simulink model "MotorXploer"  (R2025b)
settings: Solver=FixedStepAuto  StartTime=0.0  StopTime=inf  FixedStep=0.001  RelTol=1e-3  EnableMultiTasking=on
values from neighbouring files (symbols this model uses):
  bw_den = [1, A2 / A1, A3 / A1]    [Lab1_motor_params_student.m]
  bw_num = [(Km * dt2) / A1, 0, 0]    [Lab1_motor_params_student.m]
  dt = 0.01    [Lab1_motor_params_student.m]    (also in comport.m = 0.002)
  fw_den = [1, fw_termW1, fw_termW2]    [Lab1_motor_params_student.m]
  fw_num = [0, 0, fw_termV]    [Lab1_motor_params_student.m]
  motor_B = 8.84E-05    (= 8.84e-05)    [Lab1_motor_params_student.m]
  motor_B_Chirp = 4.18E-04    (= 0.000418)    [Lab1_motor_params_student.m]
  motor_B_Ramp = 1.07E-04    (= 0.000107)    [Lab1_motor_params_student.m]
  motor_B_Sin2Pi = 7.21e-05    [Lab1_motor_params_student.m]
  motor_B_SinPi = 1.55E-04    (= 0.000155)    [Lab1_motor_params_student.m]
  motor_B_SinPi_2 = 7.21E-05    (= 7.21e-05)    [Lab1_motor_params_student.m]
  motor_B_Stair = 6.12303E-05    (= 6.12303e-05)    [Lab1_motor_params_student.m]
  motor_Eff = 0.99866    [Lab1_motor_params_student.m]
  motor_Eff_Chirp = 0.992383333    [Lab1_motor_params_student.m]
  motor_Eff_Ramp = 0.973136667    [Lab1_motor_params_student.m]
  motor_Eff_Sin2Pi = 9.99e-01    (= 0.999)    [Lab1_motor_params_student.m]
  motor_Eff_SinPi = 0.99474    [Lab1_motor_params_student.m]
  motor_Eff_SinPi_2 = 0.999073333    [Lab1_motor_params_student.m]
  motor_Eff_Stair = 0.999076667    [Lab1_motor_params_student.m]
  motor_J = 1.46E-05    (= 1.46e-05)    [Lab1_motor_params_student.m]
  motor_J_Chirp = 1.12E-06    (= 1.12e-06)    [Lab1_motor_params_student.m]
  motor_J_Ramp = 0.000341863    [Lab1_motor_params_student.m]
  motor_J_Sin2Pi = 1.27e-05    [Lab1_motor_params_student.m]
  motor_J_SinPi = 1.28492E-05    (= 1.28492e-05)    [Lab1_motor_params_student.m]
  motor_J_SinPi_2 = 1.26993E-05    (= 1.26993e-05)    [Lab1_motor_params_student.m]
  motor_J_Stair = 1.35E-05    (= 1.35e-05)    [Lab1_motor_params_student.m]
  motor_Ke = 0.041524    [Lab1_motor_params_student.m]
  motor_Ke_Chirp = 0.070106333    [Lab1_motor_params_student.m]
  motor_Ke_Ramp = 0.037761333    [Lab1_motor_params_student.m]
  motor_Ke_Sin2Pi = 4.52e-02    (= 0.0452)    [Lab1_motor_params_student.m]
  motor_Ke_SinPi = 0.030033333    [Lab1_motor_params_student.m]
  motor_Ke_SinPi_2 = 0.045154    [Lab1_motor_params_student.m]
  motor_Ke_Stair = 0.044075    [Lab1_motor_params_student.m]
  motor_L = 0.002919699    [Lab1_motor_params_student.m]
  motor_R = 3.824    [Lab1_motor_params_student.m]
  tz_den = [1, B2 / B1, B3 / B1]    [Lab1_motor_params_student.m]
  tz_num = [(Km * dt2) / B1, (2 * Km * dt2) / B1, (Km * dt2) / B1]    [Lab1_motor_params_student.m]
undefined symbols (not defined in the file or in its folder): Blocking, dspblkCoreblockFVToolHelper, gcbh, LF, Non
libraries: simulink x31, amg_usbconverter_n_connect_lib x3
settings Model: Creator=beamk  LastModifiedBy=gonth
settings SolverCC: AutoInsertRateTranBlk=on
settings OptimizationCC: DefaultParameterBehavior=Inlined  EnhancedBackFolding=on  PassReuseOutputArgsAs=Individual arguments  ZeroExternalMemoryAtStartup=off  ZeroInternalMemoryAtStartup=off  MaxStackSize=64  OptimizeBlockOrder=speed  DifferentSizesBufferReuse=on  OptimizationCustomize=off  EfficientTunableParamExpr=on
settings DebuggingCC: ParameterTunabilityLossMsg=error
settings HardwareCC: ProdBitPerPointer=32.0  ProdBitPerSizeT=32.0  ProdBitPerPtrDiffT=32.0  ProdLargestAtomicInteger=Long  ProdLargestAtomicFloat=Double  ProdWordSize=32.0  ProdLongLongMode=on  ProdHWDeviceType=ARM Compatible->ARM Cortex-M
settings SFSimCC: MATLABDynamicMemAlloc=off
settings RTWCC: SystemTargetFile=ert.tlc  HardwareBoard=STM32G4xx Based  TemplateMakefile=ert_default_tmf  Toolchain=Armclang Compiler  Description=Embedded Coder
settings CodeAppCC: ForceParamTrailComments=on  IgnoreCustomStorageClasses=off  OperatorAnnotations=on  SimulinkDataObjDesc=on  SFDataObjDesc=on  InsertBlockDesc=on
settings ERTTargetCC: ExtModeTransport=3.0  ExtModeStaticAlloc=on  ExtModeStaticAllocSize=2048.0  ExtModeMexFile=ext_xcp  ExtModeIntrfLevel=Level2 - Open  TargetLangStandard=C99 (ISO)  CodeReplacementLibrary=ARM Cortex-M

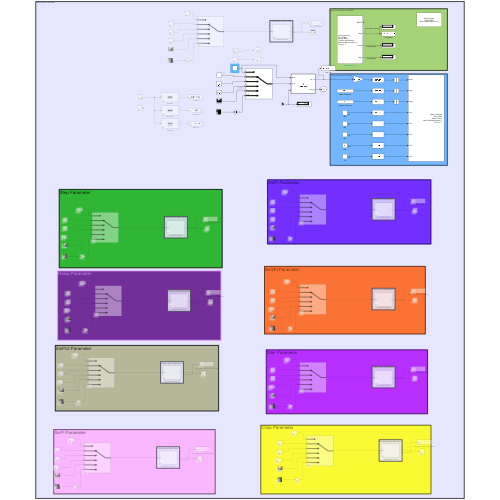
[thumbnail: Simulink's stored preview of the top-level diagram]
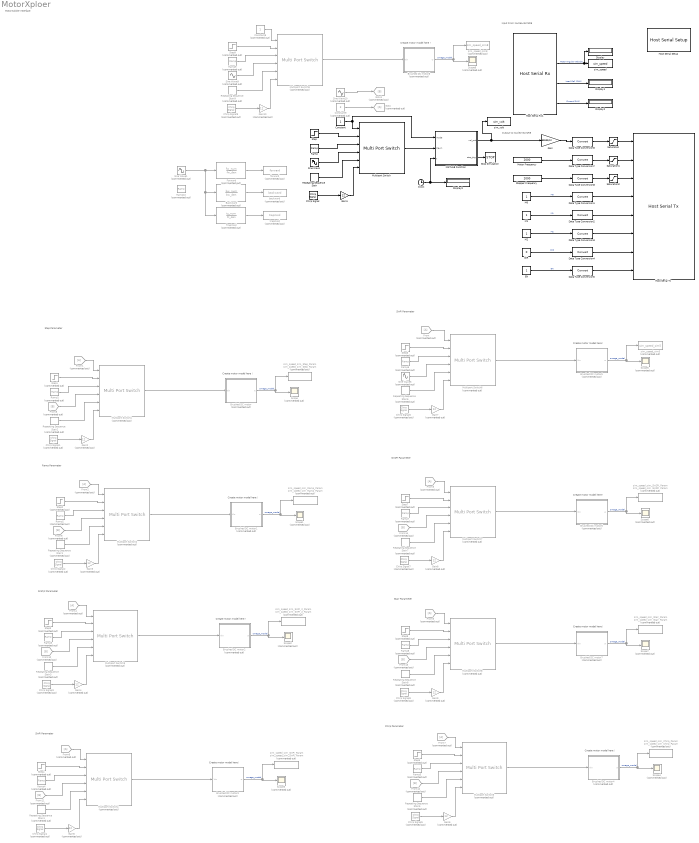
== system MotorXploer ==
  note: Output to Nucleo-G474RE
  note: Input From Nucleo-G474RE
  note: MotorXploler Interface
  note: Create motor model here !
  note: Create motor model here !
  note: Create motor model here !
  note: Create motor model here !
  note: Create motor model here !
  note: Create motor model here !
  note: Create motor model here !
  note: Create motor model here !
  note: Create motor model here !
  note: Step Parameter
  note: Ramp Parameter
  note: SinPi/2 Parameter
  note: SinPi Parameter
  note: SinPi Parameter
  note: Sin2Pi Parameter
  note: Stair Parameter
  note: Chirp Parameter
  Backward : DiscreteFilter  Commented=on  LoadFcn=dspblkCoreblockFVToolHelper(gcbh,'load');  Numerator=bw_num  Denominator=bw_den
      settings: CopyFcn=dspblkCoreblockFVToolHelper(gcbh,'copy');  DeleteFcn=dspblkCoreblockFVToolHelper(gcbh,'close');  ModelCloseFcn=dspblkCoreblockFVToolHelper(gcbh,'close');  PreSaveFcn=dspblkCoreblockFVToolHelper(gcbh,'presave');  PostSaveFcn=dspblkCoreblockFVToolHelper(gcbh,'postsave');  CloseFcn=dspblkCoreblockFVToolHelper(gcbh,'close');
  Brushed DC motor : Subsystem  Commented=on
  Brushed DC motor1 : Subsystem  Commented=on
  Brushed DC motor2 : Subsystem  Commented=on
  Brushed DC motor3 : Subsystem  Commented=on
  Brushed DC motor4 : Subsystem  Commented=on
  Brushed DC motor5 : Subsystem  Commented=on
  Brushed DC motor6 : Subsystem  Commented=on
  Brushed DC motor7 : Subsystem  Commented=on
  Brushed DC motor8 : Subsystem  Commented=on
  Chirp Signal : simulink/Sources/Chirp Signal  f1=0.1  T=30  f2=1
  Chirp Signal{1..9} (9 alike) : simulink/Sources/Chirp Signal  Commented=on  f1=0.1  T=30  f2=1
  Clock : Clock
  Constant : Constant
  Constant6 : Constant  Commented=on
  Constant9 : Constant  Commented=on  Value=3
  DIR : Constant  Value=0
  Data Type Conversion{1..8} (8 alike) : DataTypeConversion  SaturateOnIntegerOverflow=off  RndMeth=Floor
  Display{,1..3} (4 alike) : Display
  EN : Constant
  Forward : DiscreteFilter  Commented=on  LoadFcn=dspblkCoreblockFVToolHelper(gcbh,'load');  Numerator=fw_num  Denominator=fw_den
      settings: CopyFcn=dspblkCoreblockFVToolHelper(gcbh,'copy');  DeleteFcn=dspblkCoreblockFVToolHelper(gcbh,'close');  ModelCloseFcn=dspblkCoreblockFVToolHelper(gcbh,'close');  PreSaveFcn=dspblkCoreblockFVToolHelper(gcbh,'presave');  PostSaveFcn=dspblkCoreblockFVToolHelper(gcbh,'postsave');  CloseFcn=dspblkCoreblockFVToolHelper(gcbh,'close');
  From{,1..7} (8 alike) : From  Commented=on
  From{8..14} (7 alike) : From  Commented=on  GotoTag=B
  Gain : Gain  Gain=65535/12
  Gain1 : Gain  Gain=12
  Gain{2..10} (9 alike) : Gain  Commented=on  Gain=12
  Goto : Goto  Commented=on
  Goto1 : Goto  Commented=on  GotoTag=B
  Host Serial Rx1 : amg_usbconverter_n_connect_lib/Host Serial Rx  conf=rx  port=<auto>  baudrate=2000000  databits=8  parity=None  stopbit=1  flowcontrol=None  transfer=Non-Blocking  timeout=5  packetmode=Binary  enableinitialvalues=off  initialvalues=[]  binheader='25'  binterminator='4E'  porttype_double=0  porttype_single=3  porttype_int8=0  porttype_uint8=0  porttype_int16=0  porttype_uint16=0  porttype_int32=0  porttype_uint32=0  asciiformat='%f,%f,%d,%d'  rx_asciiterminator="LF (0x0A - \"\\n\")"  tx_asciiterminator="CRLF (0x0D 0x0A - \"\\r\\n\")"  sampletime=-1  enablecustomportlabel=off  cinputportlabel=0  coutputportlabel=A  portpinstr=0  blockid=HostSerialRx1  inputporttype=[]  inputportwidth=[]  inputportlabel={}  outputporttype=[3 1 1 1]  outputportwidth=[1 1 1 1]  outputportlabel={'READY','single','single','single'}  compat=0  optionstring=[]  autoport='COM5'
  Host Serial Setup : amg_usbconverter_n_connect_lib/Host Serial Setup  conf=setup  port=<auto>  baudrate=2000000  databits=8  parity=None  stopbit=1  flowcontrol=None  transfer=Blocking  timeout=2  packetmode=Binary  initialvalues=[]  binheader='7E 7E'  binterminator='03 03'  porttype_double=0  porttype_single=1  porttype_int8=0  porttype_uint8=0  porttype_int16=0  porttype_uint16=0  porttype_int32=0  porttype_uint32=2  asciiformat='%d %u %x'  rx_asciiterminator="CRLF (0x0D 0x0A - \"\\r\\n\")"  tx_asciiterminator="CRLF (0x0D 0x0A - \"\\r\\n\")"  sampletime=-1  enablecustomportlabel=off  cinputportlabel=0  coutputportlabel=A  portpinstr=0  blockid=HostSerialSetup  inputporttype=[]  inputportwidth=[]  inputportlabel={}  outputporttype=[]  outputportwidth=[]  outputportlabel={}  compat=0  optionstring=[]  autoport='COM5'
  Host Serial Tx : amg_usbconverter_n_connect_lib/Host Serial Tx  conf=tx  port=<auto>  baudrate=2000000  databits=8  parity=None  stopbit=1  flowcontrol=None  transfer=Blocking  timeout=2  packetmode=Binary  initialvalues=[]  binheader='25'  binterminator='4E'  porttype_double=0  porttype_single=3  porttype_int8=0  porttype_uint8=0  porttype_int16=5  porttype_uint16=0  porttype_int32=0  porttype_uint32=0  asciiformat='%d,%f'  rx_asciiterminator="CRLF (0x0D 0x0A - \"\\r\\n\")"  tx_asciiterminator="CRLF (0x0D 0x0A - \"\\r\\n\")"  sampletime=-1  enablecustomportlabel=off  cinputportlabel=0  coutputportlabel=A  portpinstr=0  blockid=HostSerialTx  inputporttype=[1 1 1 4 4 4 4 4]  inputportwidth=[1 1 1 1 1 1 1 1]  inputportlabel={'single','single','single','int16','int16','int16','int16','int16'}  outputporttype=[]  outputportwidth=[]  outputportlabel={}  compat=0  optionstring=[]  autoport='COM5'
      settings: SourceProductName=aMG USB Converter N
  M0 : Constant
  M1 : Constant
  M2 : Constant
  MATLAB Function : MATLAB Function  TreatAsAtomicUnit=on
  Motor Frequency : Constant  Value=2000  OutDataTypeStr=single
  Multiport Switch : MultiPortSwitch  Inputs=5  SaturateOnIntegerOverflow=off  InputSameDT=off
  Multiport Switch{1..9} (9 alike) : MultiPortSwitch  Commented=on  Inputs=5  SaturateOnIntegerOverflow=off  InputSameDT=off
  Ramp : simulink/Sources/Ramp  slope=1  start=1  InitialOutput=0
  Ramp{1..9} (9 alike) : simulink/Sources/Ramp  Commented=on  slope=.48  start=0  InitialOutput=0
  Ramp10 : simulink/Sources/Ramp  Commented=on  slope=1  start=1  InitialOutput=0
  Repeating Sequence Stair : simulink/Sources/Repeating Sequence Stair  OutValues="[0  3 0 6 0 9 0 12].'"  tsamp=2.778  OutMin=[]  OutMax=[]  OutDataTypeStr=double  OutputDataTypeScalingMode=double  OutDataType=fixdt(0,8)  ConRadixGroup=Best Precision: Vector-wise  OutScaling=2^-12
  Repeating Sequence Stair{1..9} (9 alike) : simulink/Sources/Repeating Sequence Stair  Commented=on  OutValues=[0 3 0 6 0 9 0 12].'  tsamp=2.778  OutMin=[]  OutMax=[]  OutDataTypeStr=double  OutputDataTypeScalingMode=double  OutDataType=fixdt(0,8)  ConRadixGroup=Best Precision: Vector-wise  OutScaling=2^-12
  Saturation : Saturate  UpperLimit=65535  LowerLimit=-65535
  Saturation1 : Saturate  UpperLimit=20000  LowerLimit=0
  Saturation2 : Saturate  UpperLimit=inf  LowerLimit=0
  Scope{,1..8} (9 alike) : Scope  Commented=on
      Scope settings: ActiveDisplayYMinimum=-7.4641136436048834  ActiveDisplayYMaximum=11.461850298961346
      Scope1 settings: ActiveDisplayYMinimum=-7.4641136436048834  ActiveDisplayYMaximum=11.461850298961346
      Scope2 settings: ActiveDisplayYMinimum=-7.4641136436048834  ActiveDisplayYMaximum=11.461850298961346  DataLoggingVariableName=ScopeData2
      Scope3 settings: ActiveDisplayYMinimum=-7.4641136436048834  ActiveDisplayYMaximum=11.461850298961346  DataLoggingVariableName=ScopeData3
      Scope4 settings: ActiveDisplayYMinimum=-7.4641136436048834  ActiveDisplayYMaximum=11.461850298961346  DataLoggingVariableName=ScopeData4
      Scope5 settings: ActiveDisplayYMinimum=-7.4641136436048834  ActiveDisplayYMaximum=11.461850298961346  DataLoggingVariableName=ScopeData5
      Scope6 settings: ActiveDisplayYMinimum=-7.4641136436048834  ActiveDisplayYMaximum=11.461850298961346  DataLoggingVariableName=ScopeData6
      Scope7 settings: ActiveDisplayYMinimum=-7.4641136436048834  ActiveDisplayYMaximum=11.461850298961346  DataLoggingVariableName=ScopeData7
      Scope8 settings: ActiveDisplayYMinimum=-7.4641136436048834  ActiveDisplayYMaximum=11.461850298961346  DataLoggingVariableName=ScopeData8
  Sine Wave : Sin  Amplitude=12  Frequency=pi*2  SampleTime=0
  Sine Wave1 : Sin  Commented=on  Amplitude=12  Frequency=pi*2  SampleTime=dt
  Sine Wave10 : Sin  Commented=on  Amplitude=12  Frequency=pi*2  SampleTime=0
  Sine Wave6 : Sin  Commented=on  Amplitude=12  Frequency=2*pi  SampleTime=0
  Sine Wave9 : Sin  Commented=on  Amplitude=12  Frequency=2*pi  SampleTime=0
  Step : Step  After=12  SampleTime=0
  Step{1..9} (9 alike) : Step  Commented=on  After=12  SampleTime=0
  Stepper Frequency : Constant  Value=2000  OutDataTypeStr=single
  Stop Simulation : Stop
  Trapizoid : DiscreteFilter  Commented=on  LoadFcn=dspblkCoreblockFVToolHelper(gcbh,'load');  Numerator=tz_num  Denominator=tz_den
      settings: CopyFcn=dspblkCoreblockFVToolHelper(gcbh,'copy');  DeleteFcn=dspblkCoreblockFVToolHelper(gcbh,'close');  ModelCloseFcn=dspblkCoreblockFVToolHelper(gcbh,'close');  PreSaveFcn=dspblkCoreblockFVToolHelper(gcbh,'presave');  PostSaveFcn=dspblkCoreblockFVToolHelper(gcbh,'postsave');  CloseFcn=dspblkCoreblockFVToolHelper(gcbh,'close');
  backward : ToWorkspace  Commented=on  VariableName=backward  SaveFormat=Timeseries  SampleTime=-1
  forward : ToWorkspace  Commented=on  VariableName=forward  SaveFormat=Timeseries  SampleTime=-1
  sim_speed : ToWorkspace  VariableName=sim_speed  SaveFormat=Timeseries  SampleTime=-1
  sim_speed_sim5 : ToWorkspace  Commented=on  VariableName=sim_speed_sim5  SaveFormat=Timeseries  SampleTime=-1
  sim_speed_sim8 : ToWorkspace  Commented=on  VariableName=sim_speed_sim8  SaveFormat=Timeseries  SampleTime=-1
  sim_speed_sim_Chirp_Param : ToWorkspace  Commented=on  VariableName=sim_speed_sim_Chirp_Param  SaveFormat=Timeseries  SampleTime=-1
  sim_speed_sim_Ramp_Param : ToWorkspace  Commented=on  VariableName=sim_speed_sim_Ramp_Param  SaveFormat=Timeseries  SampleTime=-1
  sim_speed_sim_Sin2Pi_Param : ToWorkspace  Commented=on  VariableName=sim_speed_sim_Sin2Pi_Param  SaveFormat=Timeseries  SampleTime=-1
  sim_speed_sim_SinPi_2_Param : ToWorkspace  Commented=on  VariableName=sim_speed_sim_SinPi_2_Param  SaveFormat=Timeseries  SampleTime=-1
  sim_speed_sim_SinPi_Param : ToWorkspace  Commented=on  VariableName=sim_speed_sim_SinPi_Param  SaveFormat=Timeseries  SampleTime=-1
  sim_speed_sim_Stair_Param : ToWorkspace  Commented=on  VariableName=sim_speed_sim_Stair_Param  SaveFormat=Timeseries  SampleTime=-1
  sim_speed_sim_Step_Param : ToWorkspace  Commented=on  VariableName=sim_speed_sim_Step_Param  SaveFormat=Timeseries  SampleTime=-1
  sim_volt : ToWorkspace  VariableName=sim_volt  SaveFormat=Timeseries  SampleTime=-1
  trapizoid : ToWorkspace  Commented=on  VariableName=trapizoid  SaveFormat=Timeseries  SampleTime=-1
  wires:
  Host Serial Rx1/2 -> sim_speed/1, Display/1  "Motor Angular Velocity"
  Host Serial Rx1/3 -> Display1/1  "Load Cell (PA0)"
  M0/1 -> Data Type Conversion1/1  "M0"
  EN/1 -> Data Type Conversion5/1  "EN"
  DIR/1 -> Data Type Conversion4/1  "DIR"
  M1/1 -> Data Type Conversion2/1  "M1"
  M2/1 -> Data Type Conversion3/1  "M2"
  Motor Frequency/1 -> Data Type Conversion7/1
  Stepper Frequency/1 -> Data Type Conversion8/1
  Data Type Conversion1/1 -> Host Serial Tx/4
  Data Type Conversion2/1 -> Host Serial Tx/5
  Data Type Conversion3/1 -> Host Serial Tx/6
  Data Type Conversion4/1 -> Host Serial Tx/7
  Data Type Conversion5/1 -> Host Serial Tx/8
  Data Type Conversion6/1 -> Saturation/1
  Saturation/1 -> Host Serial Tx/1
  Data Type Conversion7/1 -> Saturation1/1
  Data Type Conversion8/1 -> Saturation2/1
  Saturation1/1 -> Host Serial Tx/2
  Saturation2/1 -> Host Serial Tx/3
  Host Serial Rx1/4 -> Display2/1  "Current (PA1)"
  Step/1 -> Multiport Switch/2
  Constant/1 -> MATLAB Function/1(mode), Multiport Switch/1
  Ramp/1 -> Multiport Switch/3
  Sine Wave/1 -> Multiport Switch/4
  Repeating Sequence Stair/1 -> Multiport Switch/5
  Chirp Signal/1 -> Gain1/1
  Gain1/1 -> Multiport Switch/6
  Multiport Switch/1 -> MATLAB Function/2(sig_in)
  Clock/1 -> Display3/1, MATLAB Function/3(t)
  MATLAB Function/1(val_out) -> Gain/1, sim_volt/1
  MATLAB Function/2(stop_trig) -> Stop Simulation/1
  Gain/1 -> Data Type Conversion6/1
  Multiport Switch1/1 -> Brushed DC motor/1(Vin)
  From8/1 -> Multiport Switch1/4
  From1/1 -> Multiport Switch1/1
  Repeating Sequence Stair2/1 -> Multiport Switch1/5
  Step1/1 -> Multiport Switch1/2
  Gain2/1 -> Multiport Switch1/6
  Brushed DC motor/1(w) -> Scope/1, sim_speed_sim_Step_Param/1  "omega_model"
  Ramp1/1 -> Multiport Switch1/3
  Chirp Signal1/1 -> Gain2/1
  From2/1 -> Multiport Switch2/1
  Chirp Signal2/1 -> Gain3/1
  From9/1 -> Multiport Switch2/4
  Brushed DC motor1/1(w) -> Scope1/1, sim_speed_sim_Ramp_Param/1  "omega_model"
  Multiport Switch2/1 -> Brushed DC motor1/1(Vin)
  Step2/1 -> Multiport Switch2/2
  Gain3/1 -> Multiport Switch2/6
  Ramp2/1 -> Multiport Switch2/3
  Repeating Sequence Stair1/1 -> Multiport Switch2/5
  From4/1 -> Multiport Switch3/1
  Chirp Signal3/1 -> Gain4/1
  From10/1 -> Multiport Switch3/4
  Brushed DC motor2/1(w) -> Scope2/1, sim_speed_sim_SinPi_2_Param/1  "omega_model"
  Multiport Switch3/1 -> Brushed DC motor2/1(Vin)
  Step3/1 -> Multiport Switch3/2
  Gain4/1 -> Multiport Switch3/6
  Ramp3/1 -> Multiport Switch3/3
  Repeating Sequence Stair3/1 -> Multiport Switch3/5
  From6/1 -> Multiport Switch4/1
  Chirp Signal4/1 -> Gain5/1
  From11/1 -> Multiport Switch4/4
  Brushed DC motor3/1(w) -> Scope3/1, sim_speed_sim_SinPi_Param/1  "omega_model"
  Multiport Switch4/1 -> Brushed DC motor3/1(Vin)
  Step4/1 -> Multiport Switch4/2
  Gain5/1 -> Multiport Switch4/6
  Ramp4/1 -> Multiport Switch4/3
  Repeating Sequence Stair4/1 -> Multiport Switch4/5
  From7/1 -> Multiport Switch5/1
  Chirp Signal5/1 -> Gain6/1
  From12/1 -> Multiport Switch5/4
  Brushed DC motor4/1(w) -> Scope4/1, sim_speed_sim_Chirp_Param/1  "omega_model"
  Multiport Switch5/1 -> Brushed DC motor4/1(Vin)
  Step5/1 -> Multiport Switch5/2
  Gain6/1 -> Multiport Switch5/6
  Ramp5/1 -> Multiport Switch5/3
  Repeating Sequence Stair5/1 -> Multiport Switch5/5
  From/1 -> Multiport Switch6/1
  Chirp Signal6/1 -> Gain7/1
  Sine Wave6/1 -> Multiport Switch6/4
  Brushed DC motor5/1(w) -> Scope5/1, sim_speed_sim5/1  "omega_model"
  Multiport Switch6/1 -> Brushed DC motor5/1(Vin)
  Step6/1 -> Multiport Switch6/2
  Gain7/1 -> Multiport Switch6/6
  Ramp6/1 -> Multiport Switch6/3
  Repeating Sequence Stair6/1 -> Multiport Switch6/5
  From3/1 -> Multiport Switch7/1
  Chirp Signal7/1 -> Gain8/1
  From14/1 -> Multiport Switch7/4
  Brushed DC motor6/1(w) -> Scope6/1, sim_speed_sim_Sin2Pi_Param/1  "omega_model"
  Multiport Switch7/1 -> Brushed DC motor6/1(Vin)
  Step7/1 -> Multiport Switch7/2
  Gain8/1 -> Multiport Switch7/6
  Ramp7/1 -> Multiport Switch7/3
  Repeating Sequence Stair7/1 -> Multiport Switch7/5
  From5/1 -> Multiport Switch8/1
  Chirp Signal8/1 -> Gain9/1
  From13/1 -> Multiport Switch8/4
  Brushed DC motor7/1(w) -> Scope7/1, sim_speed_sim_Stair_Param/1  "omega_model"
  Multiport Switch8/1 -> Brushed DC motor7/1(Vin)
  Step8/1 -> Multiport Switch8/2
  Gain9/1 -> Multiport Switch8/6
  Ramp8/1 -> Multiport Switch8/3
  Repeating Sequence Stair8/1 -> Multiport Switch8/5
  Constant9/1 -> Goto/1
  Constant6/1 -> Multiport Switch9/1
  Chirp Signal9/1 -> Gain10/1
  Sine Wave9/1 -> Multiport Switch9/4
  Brushed DC motor8/1(w) -> Scope8/1, sim_speed_sim8/1  "omega_model"
  Multiport Switch9/1 -> Brushed DC motor8/1(Vin)
  Step9/1 -> Multiport Switch9/2
  Gain10/1 -> Multiport Switch9/6
  Ramp9/1 -> Multiport Switch9/3
  Repeating Sequence Stair9/1 -> Multiport Switch9/5
  Sine Wave10/1 -> Goto1/1
  Sine Wave1/1 -> Trapizoid/1, Backward/1, Forward/1
  Forward/1 -> forward/1
  Backward/1 -> backward/1
  Trapizoid/1 -> trapizoid/1

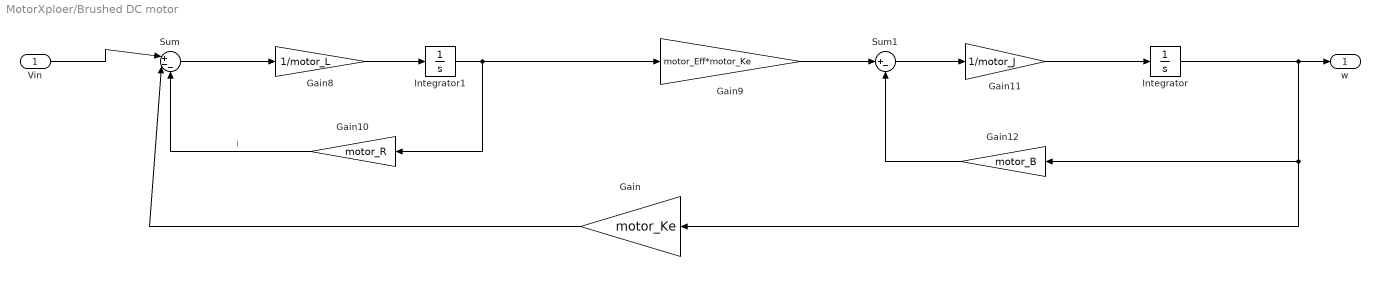
== system MotorXploer/Brushed DC motor ==
  Vin : Inport
  Gain : Gain  Gain=motor_Ke
  Gain10 : Gain  Gain=motor_R
  Gain11 : Gain  Gain=1/motor_J
  Gain12 : Gain  Gain=motor_B
  Gain8 : Gain  Gain=1/motor_L
  Gain9 : Gain  Gain=motor_Eff*motor_Ke
  Integrator : Integrator
  Integrator1 : Integrator
  Sum : Sum  Inputs=|+--
  Sum1 : Sum  Inputs=|+-
  w : Outport
  wires:
  Vin/1 -> Sum/1
  Sum/1 -> Gain8/1
  Gain8/1 -> Integrator1/1
  Integrator1/1 -> Gain9/1, Gain10/1
  Gain11/1 -> Integrator/1
  Integrator/1 -> Gain12/1, Gain/1, w/1
  Gain/1 -> Sum/2
  Gain10/1 -> Sum/3  "i"
  Gain9/1 -> Sum1/1
  Sum1/1 -> Gain11/1
  Gain12/1 -> Sum1/2

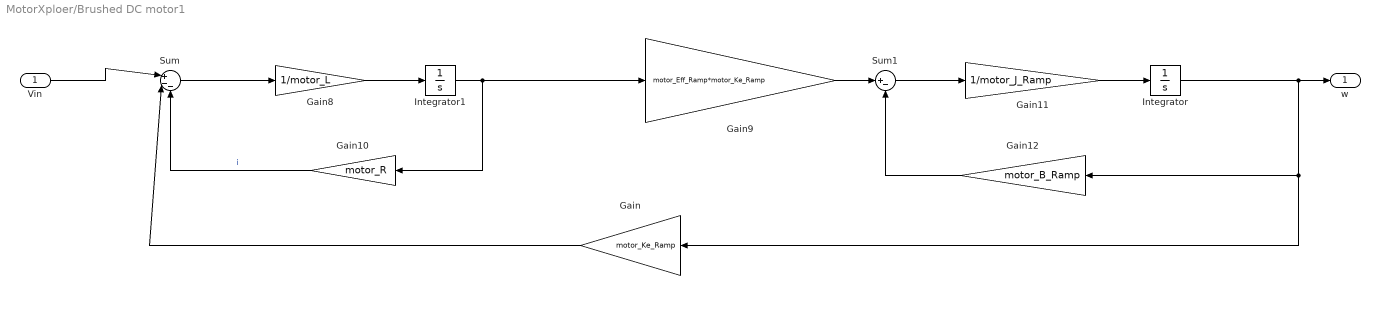
== system MotorXploer/Brushed DC motor1 ==
  Vin : Inport
  Gain : Gain  Gain=motor_Ke_Ramp
  Gain10 : Gain  Gain=motor_R
  Gain11 : Gain  Gain=1/motor_J_Ramp
  Gain12 : Gain  Gain=motor_B_Ramp
  Gain8 : Gain  Gain=1/motor_L
  Gain9 : Gain  Gain=motor_Eff_Ramp*motor_Ke_Ramp
  Integrator : Integrator
  Integrator1 : Integrator
  Sum : Sum  Inputs=|+--
  Sum1 : Sum  Inputs=|+-
  w : Outport
  wires:
  Vin/1 -> Sum/1
  Sum/1 -> Gain8/1
  Gain8/1 -> Integrator1/1
  Integrator1/1 -> Gain9/1, Gain10/1
  Gain11/1 -> Integrator/1
  Integrator/1 -> Gain/1, Gain12/1, w/1
  Gain/1 -> Sum/2
  Gain10/1 -> Sum/3  "i"
  Gain9/1 -> Sum1/1
  Sum1/1 -> Gain11/1
  Gain12/1 -> Sum1/2

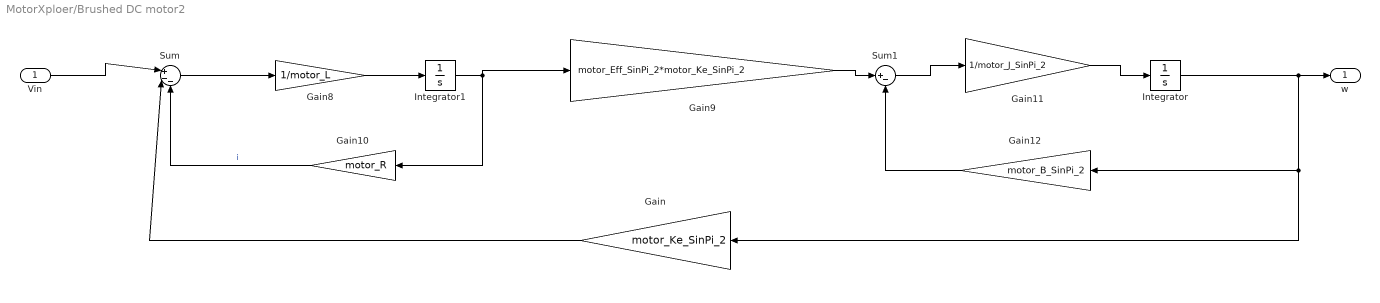
== system MotorXploer/Brushed DC motor2 ==
  Vin : Inport
  Gain : Gain  Gain=motor_Ke_SinPi_2
  Gain10 : Gain  Gain=motor_R
  Gain11 : Gain  Gain=1/motor_J_SinPi_2
  Gain12 : Gain  Gain=motor_B_SinPi_2
  Gain8 : Gain  Gain=1/motor_L
  Gain9 : Gain  Gain=motor_Eff_SinPi_2*motor_Ke_SinPi_2
  Integrator : Integrator
  Integrator1 : Integrator
  Sum : Sum  Inputs=|+--
  Sum1 : Sum  Inputs=|+-
  w : Outport
  wires:
  Vin/1 -> Sum/1
  Sum/1 -> Gain8/1
  Gain8/1 -> Integrator1/1
  Integrator1/1 -> Gain9/1, Gain10/1
  Gain11/1 -> Integrator/1
  Integrator/1 -> Gain/1, Gain12/1, w/1
  Gain/1 -> Sum/2
  Gain10/1 -> Sum/3  "i"
  Gain9/1 -> Sum1/1
  Sum1/1 -> Gain11/1
  Gain12/1 -> Sum1/2

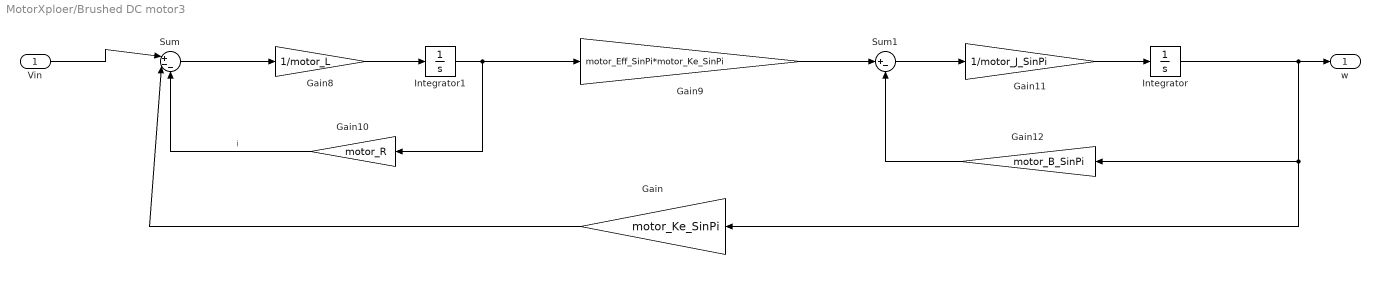
== system MotorXploer/Brushed DC motor3 ==
  Vin : Inport
  Gain : Gain  Gain=motor_Ke_SinPi
  Gain10 : Gain  Gain=motor_R
  Gain11 : Gain  Gain=1/motor_J_SinPi
  Gain12 : Gain  Gain=motor_B_SinPi
  Gain8 : Gain  Gain=1/motor_L
  Gain9 : Gain  Gain=motor_Eff_SinPi*motor_Ke_SinPi
  Integrator : Integrator
  Integrator1 : Integrator
  Sum : Sum  Inputs=|+--
  Sum1 : Sum  Inputs=|+-
  w : Outport
  wires:
  Vin/1 -> Sum/1
  Sum/1 -> Gain8/1
  Gain8/1 -> Integrator1/1
  Integrator1/1 -> Gain9/1, Gain10/1
  Gain11/1 -> Integrator/1
  Integrator/1 -> Gain12/1, Gain/1, w/1
  Gain/1 -> Sum/2
  Gain10/1 -> Sum/3  "i"
  Gain9/1 -> Sum1/1
  Sum1/1 -> Gain11/1
  Gain12/1 -> Sum1/2

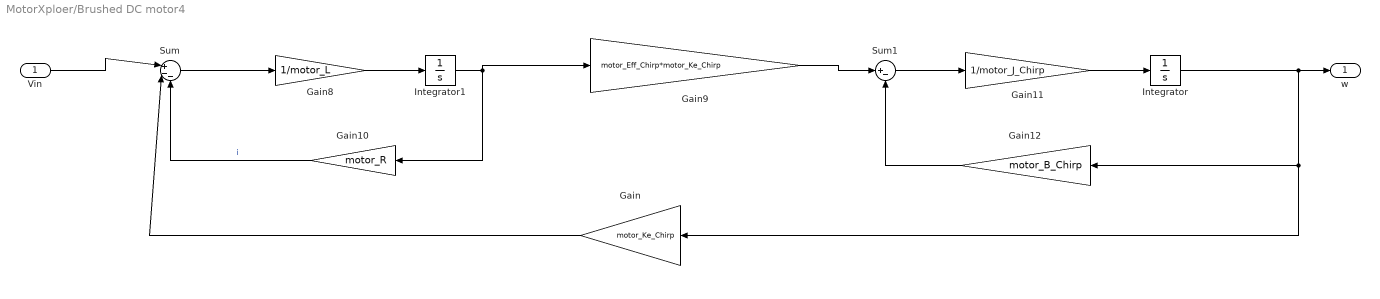
== system MotorXploer/Brushed DC motor4 ==
  Vin : Inport
  Gain : Gain  Gain=motor_Ke_Chirp
  Gain10 : Gain  Gain=motor_R
  Gain11 : Gain  Gain=1/motor_J_Chirp
  Gain12 : Gain  Gain=motor_B_Chirp
  Gain8 : Gain  Gain=1/motor_L
  Gain9 : Gain  Gain=motor_Eff_Chirp*motor_Ke_Chirp
  Integrator : Integrator
  Integrator1 : Integrator
  Sum : Sum  Inputs=|+--
  Sum1 : Sum  Inputs=|+-
  w : Outport
  wires:
  Vin/1 -> Sum/1
  Sum/1 -> Gain8/1
  Gain8/1 -> Integrator1/1
  Integrator1/1 -> Gain9/1, Gain10/1
  Gain11/1 -> Integrator/1
  Integrator/1 -> Gain/1, Gain12/1, w/1
  Gain/1 -> Sum/2
  Gain10/1 -> Sum/3  "i"
  Gain9/1 -> Sum1/1
  Sum1/1 -> Gain11/1
  Gain12/1 -> Sum1/2

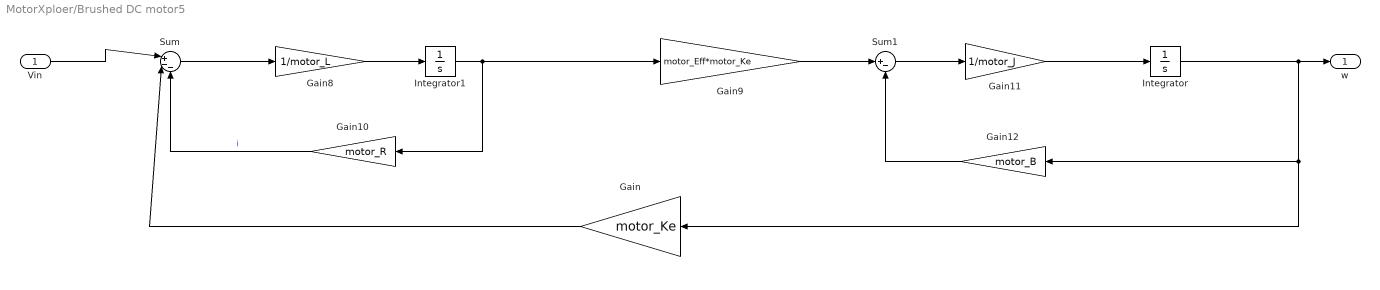
== system MotorXploer/Brushed DC motor5 ==
  Vin : Inport
  Gain : Gain  Gain=motor_Ke
  Gain10 : Gain  Gain=motor_R
  Gain11 : Gain  Gain=1/motor_J
  Gain12 : Gain  Gain=motor_B
  Gain8 : Gain  Gain=1/motor_L
  Gain9 : Gain  Gain=motor_Eff*motor_Ke
  Integrator : Integrator
  Integrator1 : Integrator
  Sum : Sum  Inputs=|+--
  Sum1 : Sum  Inputs=|+-
  w : Outport
  wires:
  Vin/1 -> Sum/1
  Sum/1 -> Gain8/1
  Gain8/1 -> Integrator1/1
  Integrator1/1 -> Gain9/1, Gain10/1
  Gain11/1 -> Integrator/1
  Integrator/1 -> Gain12/1, Gain/1, w/1
  Gain/1 -> Sum/2
  Gain10/1 -> Sum/3  "i"
  Gain9/1 -> Sum1/1
  Sum1/1 -> Gain11/1
  Gain12/1 -> Sum1/2

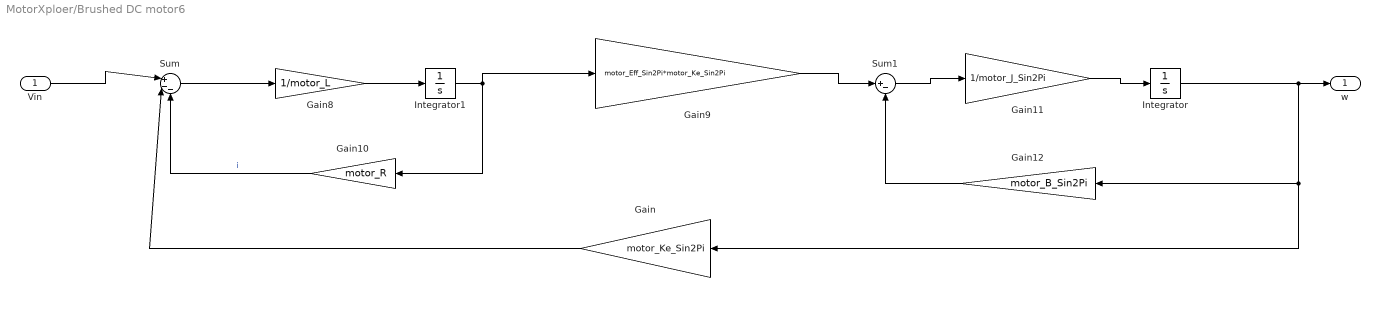
== system MotorXploer/Brushed DC motor6 ==
  Vin : Inport
  Gain : Gain  Gain=motor_Ke_Sin2Pi
  Gain10 : Gain  Gain=motor_R
  Gain11 : Gain  Gain=1/motor_J_Sin2Pi
  Gain12 : Gain  Gain=motor_B_Sin2Pi
  Gain8 : Gain  Gain=1/motor_L
  Gain9 : Gain  Gain=motor_Eff_Sin2Pi*motor_Ke_Sin2Pi
  Integrator : Integrator
  Integrator1 : Integrator
  Sum : Sum  Inputs=|+--
  Sum1 : Sum  Inputs=|+-
  w : Outport
  wires:
  Vin/1 -> Sum/1
  Sum/1 -> Gain8/1
  Gain8/1 -> Integrator1/1
  Integrator1/1 -> Gain9/1, Gain10/1
  Gain11/1 -> Integrator/1
  Integrator/1 -> Gain12/1, Gain/1, w/1
  Gain/1 -> Sum/2
  Gain10/1 -> Sum/3  "i"
  Gain9/1 -> Sum1/1
  Sum1/1 -> Gain11/1
  Gain12/1 -> Sum1/2

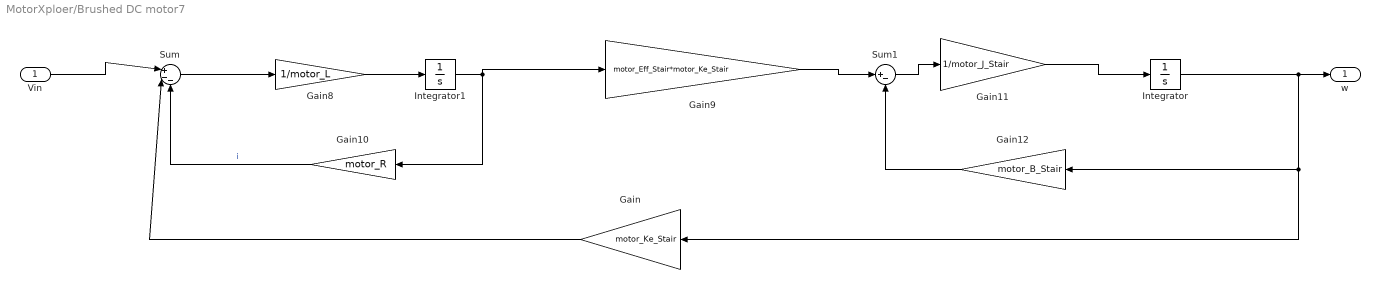
== system MotorXploer/Brushed DC motor7 ==
  Vin : Inport
  Gain : Gain  Gain=motor_Ke_Stair
  Gain10 : Gain  Gain=motor_R
  Gain11 : Gain  Gain=1/motor_J_Stair
  Gain12 : Gain  Gain=motor_B_Stair
  Gain8 : Gain  Gain=1/motor_L
  Gain9 : Gain  Gain=motor_Eff_Stair*motor_Ke_Stair
  Integrator : Integrator
  Integrator1 : Integrator
  Sum : Sum  Inputs=|+--
  Sum1 : Sum  Inputs=|+-
  w : Outport
  wires:
  Vin/1 -> Sum/1
  Sum/1 -> Gain8/1
  Gain8/1 -> Integrator1/1
  Integrator1/1 -> Gain9/1, Gain10/1
  Gain11/1 -> Integrator/1
  Integrator/1 -> Gain/1, Gain12/1, w/1
  Gain/1 -> Sum/2
  Gain10/1 -> Sum/3  "i"
  Gain9/1 -> Sum1/1
  Sum1/1 -> Gain11/1
  Gain12/1 -> Sum1/2

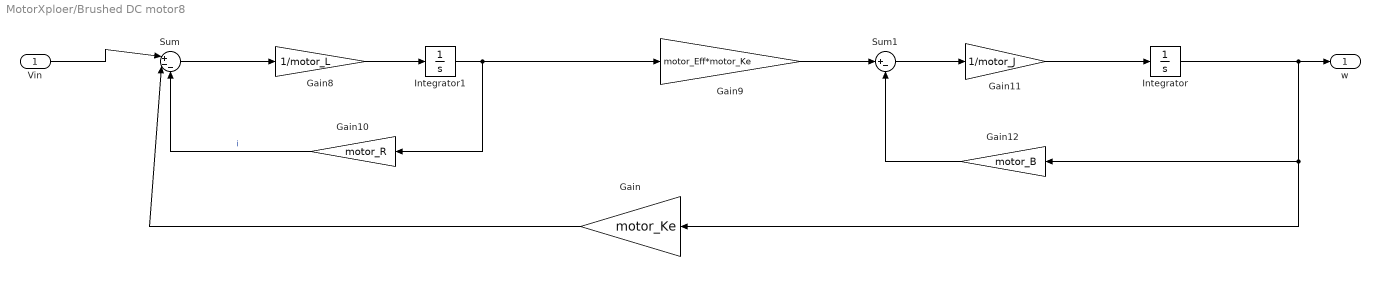
== system MotorXploer/Brushed DC motor8 ==
  Vin : Inport
  Gain : Gain  Gain=motor_Ke
  Gain10 : Gain  Gain=motor_R
  Gain11 : Gain  Gain=1/motor_J
  Gain12 : Gain  Gain=motor_B
  Gain8 : Gain  Gain=1/motor_L
  Gain9 : Gain  Gain=motor_Eff*motor_Ke
  Integrator : Integrator
  Integrator1 : Integrator
  Sum : Sum  Inputs=|+--
  Sum1 : Sum  Inputs=|+-
  w : Outport
  wires:
  Vin/1 -> Sum/1
  Sum/1 -> Gain8/1
  Gain8/1 -> Integrator1/1
  Integrator1/1 -> Gain9/1, Gain10/1
  Gain11/1 -> Integrator/1
  Integrator/1 -> Gain12/1, Gain/1, w/1
  Gain/1 -> Sum/2
  Gain10/1 -> Sum/3  "i"
  Gain9/1 -> Sum1/1
  Sum1/1 -> Gain11/1
  Gain12/1 -> Sum1/2

== matlab function MotorXploer/MATLAB Function ==
  data: mode input; sig_in input; val_out output; t input; stop_trig output
function [val_out, stop_trig] = signal_gate(mode,sig_in,  t)
    % signal_gate: คุมการจ่ายไฟ และสั่งหยุด Simulation
    % Outputs:
    %   val_out   : ค่าแรงดันส่งไปมอเตอร์
    %   stop_trig : ส่งค่า 1 ไปกระตุ้น Block 'Stop Simulation'

    % --- 1. Config เวลาของแต่ละโหมด (วินาที) ---
    % Index: 1=Step, 2=Ramp, 3=Sine, 4=Stair, 5=Chirp
    duration_list = [25, 20, 20, 25, 25]; 
    
    cooldown = 0.5; % เวลาหน่วง (วินาที) ให้กราฟตกเป็น 0 ก่อนค่อยหยุด

    % --- 2. Logic ---
    stop_trig = 0; % ค่าปกติคือยังไม่หยุด (0)
    val_out = 0;   % ค่าปกติปลอดภัยไว้ก่อน
    
    if mode >= 1 && mode <= length(duration_list)
        time_limit = duration_list(mode);
        
        if t <= time_limit
            % ช่วงทำงานปกติ: ปล่อยสัญญาณผ่าน
            val_out = sig_in;
            stop_trig = 0;
            
        elseif t <= (time_limit + cooldown)
            % ช่วง Cooldown: ตัดไฟเป็น 0 แต่ยังไม่สั่งหยุด Sim
            % (เพื่อให้เห็นกราฟตกศูนย์ใน Data Log)
            val_out = 0;
            stop_trig = 0;
            
        else
            % หมดเวลา Cooldown: ตัดไฟ และ สั่งหยุดทันที
            val_out = 0;
            stop_trig = 1; % ยิงสัญญาณหยุด!
        end
    else
        % กรณีใส่โหมดผิด
        val_out = 0;
        stop_trig = 1; 
    end
end
